simulink model "Question_3_sim"  (R2022b)
settings: Solver=VariableStepAuto  StartTime=0.0  StopTime=10.0  RelTol=1e-3
values from neighbouring files (symbols this model uses):
  b1 = 40    [Question_1_mat.m]    (also in question_3_mat.m = 36)
  b2 = 30    [Question_1_mat.m]    (also in question_3_mat.m = 26)
  g = 9.81    [Question_1_mat.m]    (also in question_3_mat.m)
  k1 = 5    [question_3_mat.m]
  k2 = 35    [question_3_mat.m]
  m1 = 2    [Question_1_mat.m]    (also in question_2_mat.m = 1; question_3_mat.m)
  m2 = 3    [Question_1_mat.m]    (also in question_2_mat.m = 1.5; question_3_mat.m)
settings Model: Creator=adnzw  LastModifiedBy=adnzw

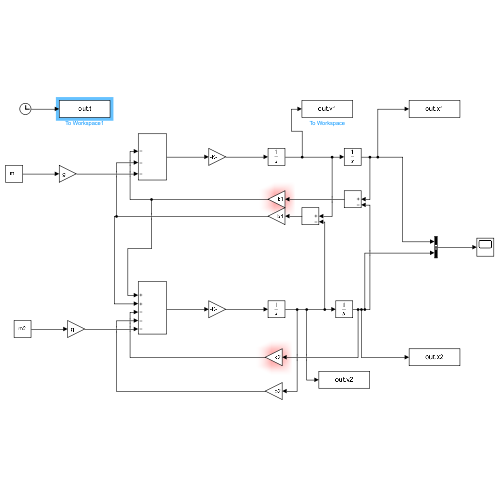
[thumbnail: Simulink's stored preview of the top-level diagram]
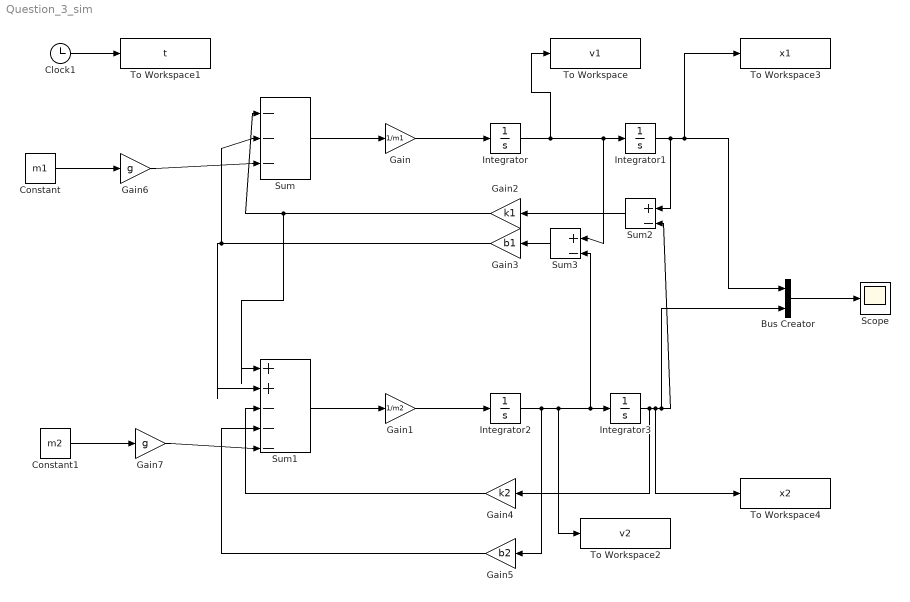
== system Question_3_sim ==
  Bus Creator : BusCreator  Inputs=2
  Clock1 : Clock
  Constant : Constant  Value=m1
  Constant1 : Constant  Value=m2
  Gain : Gain  Gain=1/m1
  Gain1 : Gain  Gain=1/m2
  Gain2 : Gain  Gain=k1
  Gain3 : Gain  Gain=b1
  Gain4 : Gain  Gain=k2
  Gain5 : Gain  Gain=b2
  Gain6 : Gain  Gain=g
  Gain7 : Gain  Gain=g
  Integrator{,1..3} (4 alike) : Integrator
  Scope : Scope
  Sum : Sum  Inputs=|---
  Sum1 : Sum  Inputs=|++---
  Sum2 : Sum  Inputs=|+-
  Sum3 : Sum  Inputs=|+-
  To Workspace : ToWorkspace  VariableName=v1  SaveFormat=Timeseries  SampleTime=-1
  To Workspace1 : ToWorkspace  VariableName=t  SaveFormat=Timeseries  SampleTime=-1
  To Workspace2 : ToWorkspace  VariableName=v2  SaveFormat=Timeseries  SampleTime=-1
  To Workspace3 : ToWorkspace  VariableName=x1  SaveFormat=Timeseries  SampleTime=-1
  To Workspace4 : ToWorkspace  VariableName=x2  SaveFormat=Timeseries  SampleTime=-1
  wires:
  Sum/1 -> Gain/1
  Sum1/1 -> Gain1/1
  Gain/1 -> Integrator/1
  Gain1/1 -> Integrator2/1
  Integrator2/1 -> Gain5/1, To Workspace2/1, Sum3/2, Integrator3/1
  Integrator/1 -> To Workspace/1, Sum3/1, Integrator1/1
  Integrator1/1 -> To Workspace3/1, Bus Creator/1, Sum2/1
  Integrator3/1 -> Gain4/1, To Workspace4/1, Bus Creator/2, Sum2/2
  Sum2/1 -> Gain2/1
  Gain2/1 -> Sum1/1, Sum/1
  Sum3/1 -> Gain3/1
  Gain3/1 -> Sum1/2, Sum/2
  Gain4/1 -> Sum1/3
  Gain5/1 -> Sum1/4
  Constant1/1 -> Gain7/1
  Gain7/1 -> Sum1/5
  Constant/1 -> Gain6/1
  Gain6/1 -> Sum/3
  Bus Creator/1 -> Scope/1
  Clock1/1 -> To Workspace1/1
